simulink model "WhiteBlancing_using_Intensity_Values_of_Background"  (R2016a)
settings: Solver=VariableStepAuto  StartTime=0.0  StopTime=10.0  RelTol=1e-3
undefined symbols (not defined in the file): Rec, SDTV
libraries: visionconversions x2, visionsources x2, visionsinks x2
settings Model: Creator=YASARA  LastModifiedBy=YASARA

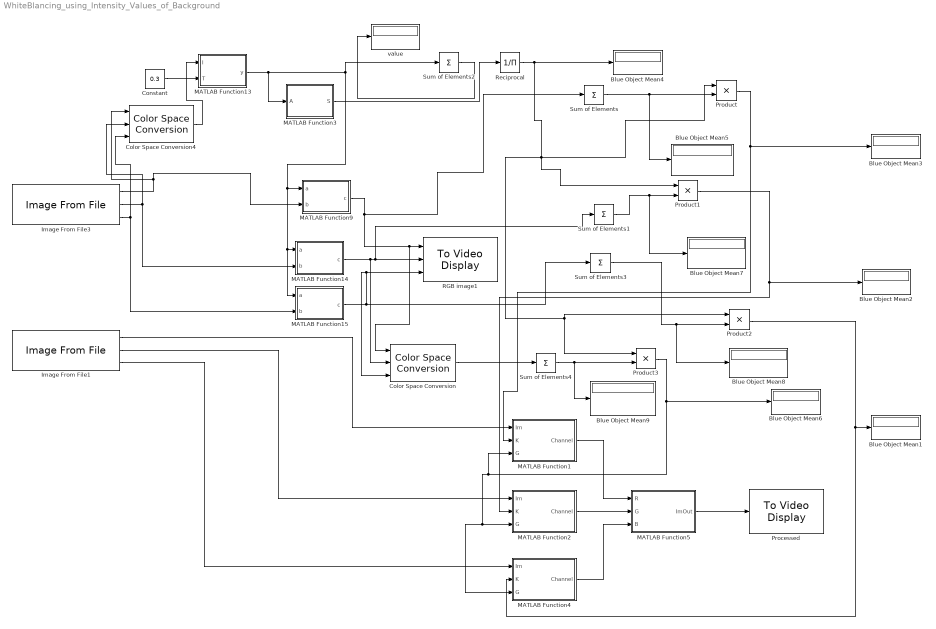
== system WhiteBlancing_using_Intensity_Values_of_Background ==
  Blue Object Mean{1..9} (9 alike) : Display
  Color Space Conversion : visionconversions/Color Space  Conversion  conversion=Obsolete  conversionActive=R'G'B' to intensity  wp_str=D65  rec=Rec. 601 (SDTV)  sys=1125/60/2:1  imagePorts=Separate color signals
  Color Space Conversion4 : visionconversions/Color Space  Conversion  conversion=Obsolete  conversionActive=R'G'B' to intensity  wp_str=D65  rec=Rec. 601 (SDTV)  sys=1125/60/2:1  imagePorts=Separate color signals
  Constant : Constant  Value=0.3  SampleTime=1
  Image From File1 : visionsources/Image From File  Tag=vipblks_nd  FileName=C:\Users\YASARA\Desktop\F1.jpg  imagePorts=Separate color signals  Ts=1  ImageDataType=uint8  Signed=on  WordLength=16  sdImageDataType=uint(8)  FractionLengthMode=User-defined  FractionLength=15  OutPortLabels=R|G|B
  Image From File3 : visionsources/Image From File  Tag=vipblks_nd  FileName=C:\Users\YASARA\Desktop\F1.jpg  imagePorts=Separate color signals  Ts=1  ImageDataType=double  Signed=on  WordLength=16  sdImageDataType=uint(8)  FractionLengthMode=User-defined  FractionLength=15  OutPortLabels=R|G|B
  MATLAB Function1 : MATLAB Function  TreatAsAtomicUnit=on
  MATLAB Function13 : MATLAB Function  TreatAsAtomicUnit=on
  MATLAB Function14 : MATLAB Function  TreatAsAtomicUnit=on
  MATLAB Function15 : MATLAB Function  TreatAsAtomicUnit=on
  MATLAB Function2 : MATLAB Function  TreatAsAtomicUnit=on
  MATLAB Function3 : MATLAB Function  TreatAsAtomicUnit=on
  MATLAB Function4 : MATLAB Function  TreatAsAtomicUnit=on
  MATLAB Function5 : MATLAB Function  TreatAsAtomicUnit=on
  MATLAB Function9 : MATLAB Function  TreatAsAtomicUnit=on
  Processed : visionsinks/To Video Display  windowSizeMode=Normal  openAtMdlStart=on  fullScreen=off  videoWindowX=252  videoWindowY=213  saveWindowSize=off  videoWindowWidth=512  videoWindowHeight=384  inputColorFormat=RGB  inputType=Obsolete  imagePorts=One multidimensional signal  OutputDevice=On-screen video monitor  dataOrg=Column-major  isWindowOpen=off
  Product{,1..3} (4 alike) : Product  OutDataTypeStr=uint8
  RGB image1 : visionsinks/To Video Display  windowSizeMode=Normal  openAtMdlStart=on  fullScreen=off  videoWindowX=252  videoWindowY=213  saveWindowSize=off  videoWindowWidth=512  videoWindowHeight=384  inputColorFormat=RGB  inputType=Obsolete  imagePorts=Separate color signals  OutputDevice=On-screen video monitor  dataOrg=Column-major  isWindowOpen=off
  Reciprocal : Product  Inputs=/  OutDataTypeStr=double  SaturateOnIntegerOverflow=on  RndMeth=Zero
  Sum of Elements{,1..4} (5 alike) : Sum  Inputs=+
  value : Display
  wires:
  Color Space Conversion4/1 -> MATLAB Function13/1(I)
  MATLAB Function9/1(c) -> Color Space Conversion/1, RGB image1/1, Sum of Elements/1
  MATLAB Function14/1(c) -> RGB image1/2, Sum of Elements1/1, Color Space Conversion/2
  MATLAB Function15/1(c) -> Sum of Elements3/1, RGB image1/3, Color Space Conversion/3
  Constant/1 -> MATLAB Function13/2(T)
  Reciprocal/1 -> Product1/1, Product3/1, Product2/1, Product/1, Blue Object Mean4/1
  MATLAB Function13/1(y) -> MATLAB Function3/1(A), MATLAB Function15/1(a), MATLAB Function14/1(a), MATLAB Function9/1(a), Sum of Elements2/1
  Image From File3/1 -> MATLAB Function9/2(b), Color Space Conversion4/1
  Image From File3/2 -> MATLAB Function14/2(b), Color Space Conversion4/2
  Image From File3/3 -> MATLAB Function15/2(b), Color Space Conversion4/3
  Image From File1/1 -> MATLAB Function1/1(Im)
  Image From File1/2 -> MATLAB Function2/1(Im)
  Image From File1/3 -> MATLAB Function4/1(Im)
  Product/1 -> MATLAB Function1/2(K), Blue Object Mean3/1
  Product1/1 -> Blue Object Mean2/1, MATLAB Function2/2(K)
  Product2/1 -> MATLAB Function4/2(K), Blue Object Mean1/1
  Color Space Conversion/1 -> Sum of Elements4/1
  Sum of Elements/1 -> Blue Object Mean5/1, Product/2
  Product3/1 -> Blue Object Mean6/1, MATLAB Function4/3(G), MATLAB Function2/3(G), MATLAB Function1/3(G)
  Sum of Elements1/1 -> Blue Object Mean7/1, Product1/2
  Sum of Elements3/1 -> Blue Object Mean8/1, Product2/2
  Sum of Elements4/1 -> Blue Object Mean9/1, Product3/2
  Sum of Elements2/1 -> value/1
  MATLAB Function3/1(S) -> Reciprocal/1
  MATLAB Function2/1(Channel) -> MATLAB Function5/2(G)
  MATLAB Function4/1(Channel) -> MATLAB Function5/3(B)
  MATLAB Function5/1(ImOut) -> Processed/1
  MATLAB Function1/1(Channel) -> MATLAB Function5/1(R)

== matlab function WhiteBlancing_using_Intensity_Values_of_Background/MATLAB Function1 ==
  data: Im input; K input; Channel output; G input
function Channel = fcn(Im,K,G)
Channel = uint8(double(Im) *double(G)/double(K));
return

== matlab function WhiteBlancing_using_Intensity_Values_of_Background/MATLAB Function2 ==
  data: Im input; K input; Channel output; G input
function Channel = fcn(Im,K,G)
Channel = uint8(double(Im) *double(G)/double(K));
return

== matlab function WhiteBlancing_using_Intensity_Values_of_Background/MATLAB Function3 ==
  data: A input; S output
function S = fcn(A)
%#codegen
S = sum(A(:))/100;

== matlab function WhiteBlancing_using_Intensity_Values_of_Background/MATLAB Function4 ==
  data: Im input; K input; Channel output; G input
function Channel = fcn(Im,K,G)
Channel = uint8(double(Im) *double(G)/double(K));
return

== matlab function WhiteBlancing_using_Intensity_Values_of_Background/MATLAB Function5 ==
  data: R input; G input; B input; ImOut output
function ImOut = fcn(R,G,B)
ImOut = cat(3, R, G, B);
return

== matlab function WhiteBlancing_using_Intensity_Values_of_Background/MATLAB Function14 ==
  data: a input; b input; c output
function c = fcn(a,b)
%#codegen
c=a.*b;
return

== matlab function WhiteBlancing_using_Intensity_Values_of_Background/MATLAB Function13 ==
  data: I input; y output; T input
function y = fcn(I,T)
%#codegen
BW = imbinarize(I,T);
y = BW;

== matlab function WhiteBlancing_using_Intensity_Values_of_Background/MATLAB Function15 ==
  data: a input; b input; c output
function c = fcn(a,b)
%#codegen
c=a.*b;
return

== matlab function WhiteBlancing_using_Intensity_Values_of_Background/MATLAB Function9 ==
  data: a input; b input; c output
function c = fcn(a,b)
%#codegen
c=a.*b;
return
